simulink model "WP_"  (R2023b)
settings: Solver=VariableStepAuto  StartTime=0.0  StopTime=40  RelTol=1e-3
settings Model: Creator=91996  LastModifiedBy=Dell

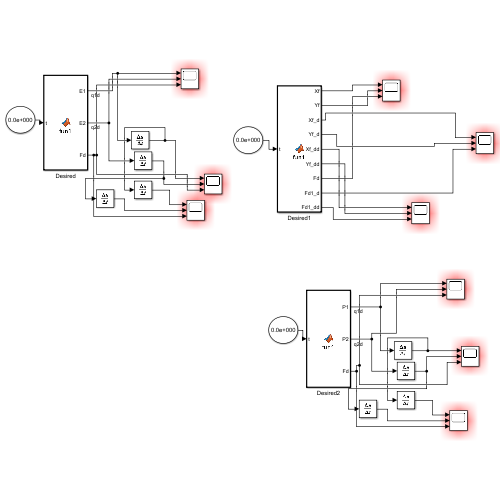
[thumbnail: Simulink's stored preview of the top-level diagram]
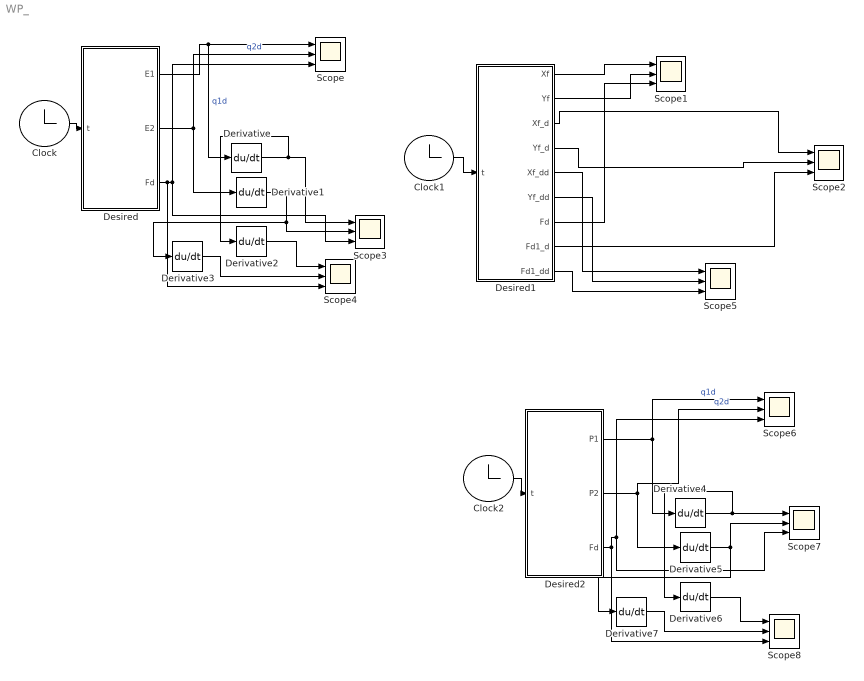
== system WP_ ==
  Clock : Clock
  Clock1 : Clock
  Clock2 : Clock
  Derivative{,1..7} (8 alike) : Derivative
  Desired : MATLAB Function  TreatAsAtomicUnit=on
  Desired1 : MATLAB Function  TreatAsAtomicUnit=on
  Desired2 : MATLAB Function  TreatAsAtomicUnit=on
  Scope{,1..8} (9 alike) : Scope  NumInputPorts=3
  wires:
  Clock/1 -> Desired/1(t)
  Desired/1(E1) -> Scope/1, Derivative/1  "q1d"
  Desired/2(E2) -> Derivative1/1, Scope/2  "q2d"
  Clock1/1 -> Desired1/1("t ")
  Desired1/3(Xf_d) -> Scope2/1
  Desired1/4(Yf_d) -> Scope2/2
  Desired1/5(Xf_dd) -> Scope5/1
  Desired1/6(Yf_dd) -> Scope5/2
  Desired1/7(Fd) -> Scope1/3
  Desired1/8(Fd1_d) -> Scope2/3
  Desired1/9(Fd1_dd) -> Scope5/3
  Desired1/1(Xf) -> Scope1/1
  Desired1/2(Yf) -> Scope1/2
  Derivative1/1 -> Derivative3/1, Scope3/2
  Derivative2/1 -> Scope4/1
  Derivative3/1 -> Scope4/2
  Desired/3(Fd) -> Scope4/3, Scope/3, Scope3/3
  Derivative/1 -> Derivative2/1, Scope3/1
  Desired2/3(Fd) -> Scope6/3, Scope7/3, Scope8/3
  Derivative7/1 -> Scope8/2
  Derivative6/1 -> Scope8/1
  Derivative5/1 -> Derivative7/1, Scope7/2
  Derivative4/1 -> Derivative6/1, Scope7/1
  Desired2/1(P1) -> Scope6/1, Derivative4/1  "q1d"
  Desired2/2(P2) -> Scope6/2, Derivative5/1  "q2d"
  Clock2/1 -> Desired2/1(t)

== matlab function WP_/Desired ==
  data: E1 output; E2 output; t input; Fd output
function [E1,E2,Fd]=fun1(t)
Yf=0.3;
Xf=0.5-0.1+0.25;
P=[Xf;Yf];
Z0=[0.1,0.2]';
h=0.0001;
L01=0.5;
L1=0.5;
L2=L1;
for jn=1:100
    t1=Z0(1);
    t2=Z0(2);
E=R_EQ(L01,L1,L2,t1,t2-0.1)-P;
Et1=R_EQ(L01,L1,L2,t1+h,t2-0.1)-P;
Et2=R_EQ(L01,L1,L2,t1,t2+h-0.1)-P;
J=([Et1 Et2]-[E E])/h;
Z1=Z0-inv(J)*E;
err=abs(Z1-Z0);
if err<=0.0001;
    break;
else
    Z0=Z1;
end
end
t1s=wrapToPi(t1);
t2s=wrapToPi(t2);
ts=40;
t10=0;
t20=-0.1;
t10_d=0;
t20_d=0;
t10_dd=0;
t20_dd=0;
[t1d,t1d_d,t1d_dd]=para_(t10,t10_d,t10_dd,t,ts,t1s);
[t2d,t2d_d,t2d_dd]=para_(t20,t20_d,t20_dd,t,ts,t2s);
Jac = R_Jac1(L1,L2,t1d,t2d-0.1);
Jd = R_Jd1(L1,L2,t1d,t2d-0.1,t1d_d,t2d_d);
PP=R_EQ(L01,L1,L2,t1d,t2d-0.1);
E1=PP(1);
E2=PP(2);
Fd=0;

== matlab function WP_/Desired2 ==
  data: P1 output; P2 output; t input; Fd output
function [P1,P2,Fd]=fun1(t)
% function [PP,Pdd,Fd]=fun1(t)

Yf0=0.3;
Yf0_d=0;
Yf0_dd=0;
Xf=0.5-0.1+0.25;

Yfs=0.2;
ts=40;
[Yf,Yf_d,Yf_dd]=para_(Yf0,Yf0_d,Yf0_dd,t,ts,Yfs);
PP=[Xf;Yf];
P1=PP(1);
P2=PP(2);
Fd=0;

== matlab function WP_/Desired1 ==
  data: Xf output; Yf output; t input; Xf_d output; Yf_d output; Xf_dd output; Yf_dd output; Fd output; Fd1_d output; Fd1_dd output
function [Xf,Yf,Xf_d,Yf_d,Xf_dd,Yf_dd,Fd,Fd1_d,Fd1_dd]=fun1(t)
% function [PP,Pdd,Fd]=fun1(t)

Yf=0.2;
% Xf0=0.5-0.1+0.25+0.01;
Xf0=0.5-0.1+0.25;
Xfs=Xf0+0.2;
Xf0_d=0;
Xf0_dd=0;
ts=40;
[Xf,Xf_d,Xf_dd]=para_(Xf0,Xf0_d,Xf0_dd,t,ts,Xfs);
PP=[Xf;Yf];
Pd=[Xf_d;0];
Pdd=[Xf_dd;0];
Yf_d=0;
Yf_dd=0;
% Fd=0.0000010;
% Fd=0.010;
Fd1s=0.15;

Fd10=0.1;
Fd10_d=0;
Fd10_dd=0;

[Fd,Fd1_d,Fd1_dd]=para_(Fd10,Fd10_d,Fd10_dd,t,ts,Fd1s);
